simulink model "bo1808_fig1_9_modular"  (R2024b)
settings: Solver=ode23tb  StartTime=0.0  StopTime=t_stop_open_loop  MaxStep=1e-5  RelTol=1e-3
model workspace (MAT data in the model file):
  B = 5.1285732711e-07
  Id_max = 0.6
  Iq_max = 0.6
  J = 1.4e-07
  Ld = 0.00037
  Lq = 0.00037
  Rs = 7.2
  TL_nom = 0.0012
  TL_step_time = 0.04
  Vdc = 11.4
  Vdq_max = 6.58179306876
  id0 = 0
  iq0 = 0
  omega_m0 = 0
  pn = 4
  psi_f = 0.00106666666667
  t_stop_open_loop = 0.08
  theta_e0 = 0
  ud_step_value = 0
  uq_step_value = 1
settings Model: Creator=26683  LastModifiedBy=26683

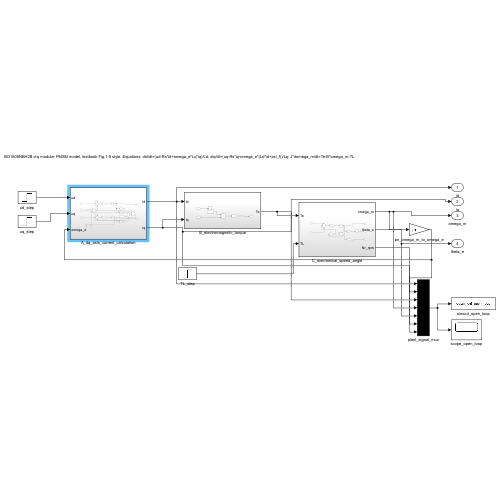
[thumbnail: Simulink's stored preview of the top-level diagram]
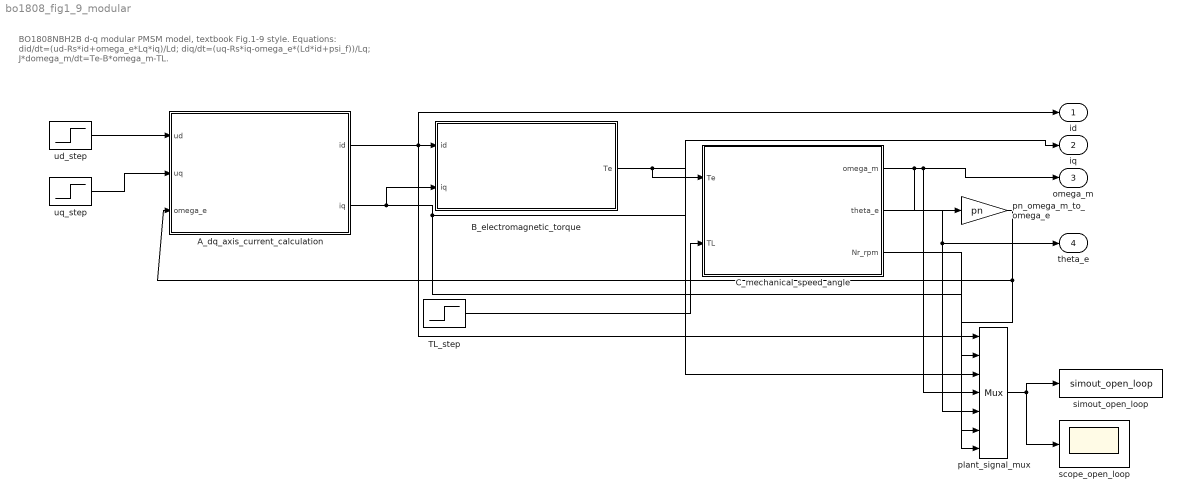
== system bo1808_fig1_9_modular ==
  note: BO1808NBH2B d-q modular PMSM model, textbook Fig.1-9 style. Equations: did/dt=(ud-Rs*id+omega_e*Lq*iq)/Ld; diq/dt=(uq-Rs*iq-omega_e*(Ld*id+psi_f))/Lq; J*domega_m/dt=Te-B*omega_m-TL.
  A_dq_axis_current_calculation : Subsystem
  B_electromagnetic_torque : Subsystem
  C_mechanical_speed_angle : Subsystem
  TL_step : Step  Time=TL_step_time  After=TL_nom  SampleTime=0
  plant_signal_mux : Mux  Inputs=7
  pn_omega_m_to_omega_e : Gain  Gain=pn
  scope_open_loop : Scope
  simout_open_loop : ToWorkspace  VariableName=simout_open_loop  SaveFormat=Structure With Time  SampleTime=-1
  ud_step : Step  Time=0.005  After=ud_step_value  SampleTime=0
  uq_step : Step  Time=0.005  After=uq_step_value  SampleTime=0
  id : Outport
  iq : Outport  Port=2
  omega_m : Outport  Port=3
  theta_e : Outport  Port=4
  wires:
  ud_step/1 -> A_dq_axis_current_calculation/1(ud)
  uq_step/1 -> A_dq_axis_current_calculation/2(uq)
  pn_omega_m_to_omega_e/1 -> A_dq_axis_current_calculation/3(omega_e), plant_signal_mux/7
  A_dq_axis_current_calculation/1(id) -> B_electromagnetic_torque/1(id), plant_signal_mux/1, id/1
  A_dq_axis_current_calculation/2(iq) -> plant_signal_mux/2, iq/1, B_electromagnetic_torque/2(iq)
  B_electromagnetic_torque/1(Te) -> C_mechanical_speed_angle/1(Te), plant_signal_mux/3
  TL_step/1 -> C_mechanical_speed_angle/2(TL)
  C_mechanical_speed_angle/1(omega_m) -> plant_signal_mux/4, omega_m/1, pn_omega_m_to_omega_e/1
  C_mechanical_speed_angle/2(theta_e) -> plant_signal_mux/5, theta_e/1
  C_mechanical_speed_angle/3(Nr_rpm) -> plant_signal_mux/6
  plant_signal_mux/1 -> simout_open_loop/1, scope_open_loop/1

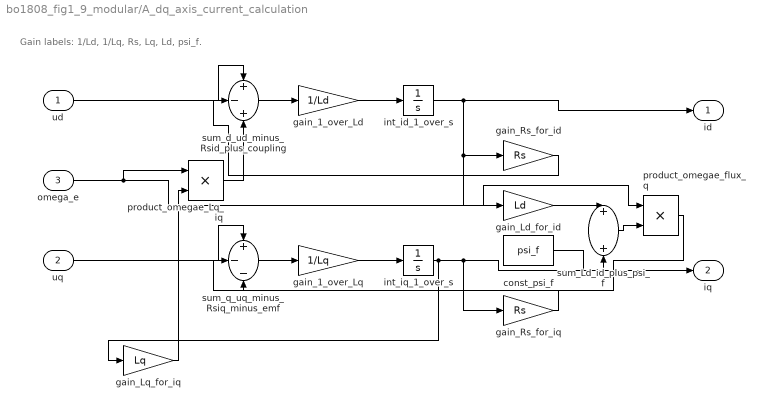
== system bo1808_fig1_9_modular/A_dq_axis_current_calculation ==
  note: Gain labels: 1/Ld, 1/Lq, Rs, Lq, Ld, psi_f.
  ud : Inport
  uq : Inport  Port=2
  omega_e : Inport  Port=3
  const_psi_f : Constant  Value=psi_f
  gain_1_over_Ld : Gain  Gain=1/Ld
  gain_1_over_Lq : Gain  Gain=1/Lq
  gain_Ld_for_id : Gain  Gain=Ld
  gain_Lq_for_iq : Gain  Gain=Lq
  gain_Rs_for_id : Gain  Gain=Rs
  gain_Rs_for_iq : Gain  Gain=Rs
  int_id_1_over_s : Integrator  InitialCondition=id0
  int_iq_1_over_s : Integrator  InitialCondition=iq0
  product_omegae_Lq_iq : Product  Inputs=**
  product_omegae_flux_q : Product  Inputs=**
  sum_Ld_id_plus_psi_f : Sum
  sum_d_ud_minus_Rsid_plus_coupling : Sum  Inputs=+-+
  sum_q_uq_minus_Rsiq_minus_emf : Sum  Inputs=+--
  id : Outport
  iq : Outport  Port=2
  wires:
  ud/1 -> sum_d_ud_minus_Rsid_plus_coupling/1
  sum_d_ud_minus_Rsid_plus_coupling/1 -> gain_1_over_Ld/1
  gain_1_over_Ld/1 -> int_id_1_over_s/1
  int_id_1_over_s/1 -> gain_Rs_for_id/1, gain_Ld_for_id/1, id/1
  gain_Rs_for_id/1 -> sum_d_ud_minus_Rsid_plus_coupling/2
  omega_e/1 -> product_omegae_Lq_iq/1, product_omegae_flux_q/1
  int_iq_1_over_s/1 -> iq/1, gain_Rs_for_iq/1, gain_Lq_for_iq/1
  gain_Lq_for_iq/1 -> product_omegae_Lq_iq/2
  product_omegae_Lq_iq/1 -> sum_d_ud_minus_Rsid_plus_coupling/3
  uq/1 -> sum_q_uq_minus_Rsiq_minus_emf/1
  sum_q_uq_minus_Rsiq_minus_emf/1 -> gain_1_over_Lq/1
  gain_1_over_Lq/1 -> int_iq_1_over_s/1
  gain_Rs_for_iq/1 -> sum_q_uq_minus_Rsiq_minus_emf/2
  gain_Ld_for_id/1 -> sum_Ld_id_plus_psi_f/1
  const_psi_f/1 -> sum_Ld_id_plus_psi_f/2
  sum_Ld_id_plus_psi_f/1 -> product_omegae_flux_q/2
  product_omegae_flux_q/1 -> sum_q_uq_minus_Rsiq_minus_emf/3

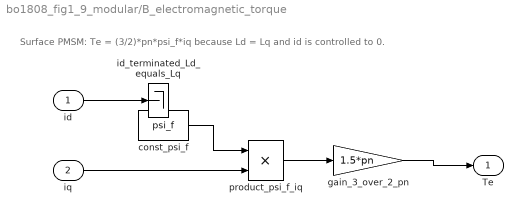
== system bo1808_fig1_9_modular/B_electromagnetic_torque ==
  note: Surface PMSM: Te = (3/2)*pn*psi_f*iq because Ld = Lq and id is controlled to 0.
  id : Inport
  iq : Inport  Port=2
  const_psi_f : Constant  Value=psi_f
  gain_3_over_2_pn : Gain  Gain=1.5*pn
  id_terminated_Ld_equals_Lq : Terminator
  product_psi_f_iq : Product  Inputs=**
  Te : Outport
  wires:
  id/1 -> id_terminated_Ld_equals_Lq/1
  const_psi_f/1 -> product_psi_f_iq/1
  iq/1 -> product_psi_f_iq/2
  product_psi_f_iq/1 -> gain_3_over_2_pn/1
  gain_3_over_2_pn/1 -> Te/1

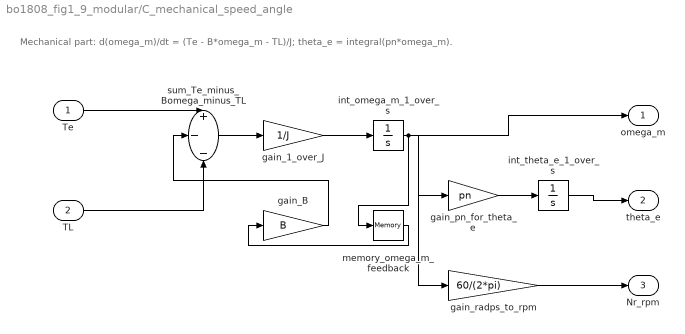
== system bo1808_fig1_9_modular/C_mechanical_speed_angle ==
  note: Mechanical part: d(omega_m)/dt = (Te - B*omega_m - TL)/J; theta_e = integral(pn*omega_m).
  Te : Inport
  TL : Inport  Port=2
  gain_1_over_J : Gain  Gain=1/J
  gain_B : Gain  Gain=B
  gain_pn_for_theta_e : Gain  Gain=pn
  gain_radps_to_rpm : Gain  Gain=60/(2*pi)
  int_omega_m_1_over_s : Integrator  InitialCondition=omega_m0
  int_theta_e_1_over_s : Integrator  InitialCondition=theta_e0
  memory_omega_m_feedback : Memory
  sum_Te_minus_Bomega_minus_TL : Sum  Inputs=+--
  omega_m : Outport
  theta_e : Outport  Port=2
  Nr_rpm : Outport  Port=3
  wires:
  Te/1 -> sum_Te_minus_Bomega_minus_TL/1
  TL/1 -> sum_Te_minus_Bomega_minus_TL/3
  sum_Te_minus_Bomega_minus_TL/1 -> gain_1_over_J/1
  gain_1_over_J/1 -> int_omega_m_1_over_s/1
  int_omega_m_1_over_s/1 -> omega_m/1, memory_omega_m_feedback/1, gain_pn_for_theta_e/1, gain_radps_to_rpm/1
  memory_omega_m_feedback/1 -> gain_B/1
  gain_B/1 -> sum_Te_minus_Bomega_minus_TL/2
  gain_pn_for_theta_e/1 -> int_theta_e_1_over_s/1
  int_theta_e_1_over_s/1 -> theta_e/1
  gain_radps_to_rpm/1 -> Nr_rpm/1
